simulink model "mcb_pmsm_foc_sensorless_dyno_f28379d"  (R2024b)
settings: Solver=FixedStepDiscrete  StartTime=0.0  StopTime=6  RelTol=1e-3  EnableMultiTasking=on
InitFcn:
  | mcb_pmsm_foc_sensorless_dyno_f28379d_datascript;
model workspace (MAT data in the model file):
  encoderResolution = 2000
  hallOffset = '0.5'
  indexOffset = 850
  polePairs = '4'
values from neighbouring files (symbols this model uses):
  acceleration = 20000/PU_System_motor1.N_base    [mcb_pmsm_foc_sensorless_dyno_f28379d_datascript.m]    (also in soc_mcb_pmsm_foc_dyno_f28379d_data.m = 20000/PU_System.N_base)
  dataType = 'single'    [mcb_pmsm_foc_sensorless_dyno_f28379d_datascript.m]    (also in soc_mcb_pmsm_foc_dyno_f28379d_data.m)
  inverter_motor1 = mcb_SetInverterParameters('BoostXL-DRV8305')    [mcb_pmsm_foc_sensorless_dyno_f28379d_datascript.m]
  inverter_motor2 = mcb_SetInverterParameters('BoostXL-DRV8305')    [mcb_pmsm_foc_sensorless_dyno_f28379d_datascript.m]
  PI_params_motor1 = mcb.internal.SetControllerParameters(pmsm_motor1,inverter_motor1,PU_System_motor1,T_pwm,2*Ts,Ts_speed)    [mcb_pmsm_foc_sensorless_dyno_f28379d_datascript.m]
  PI_params_motor2 = mcb.internal.SetControllerParameters(pmsm_motor2,inverter_motor2,PU_System_motor2,T_pwm,2*Ts,Ts_speed)    [mcb_pmsm_foc_sensorless_dyno_f28379d_datascript.m]
  pmsm_motor1 = mcb_SetPMSMMotorParameters('Teknic2310P')    [mcb_pmsm_foc_sensorless_dyno_f28379d_datascript.m]
  pmsm_motor2 = mcb_SetPMSMMotorParameters('Teknic2310P')    [mcb_pmsm_foc_sensorless_dyno_f28379d_datascript.m]
  PU_System_motor1 = mcb_SetPUSystem(pmsm_motor1,inverter_motor1)    [mcb_pmsm_foc_sensorless_dyno_f28379d_datascript.m]
  PU_System_motor2 = mcb_SetPUSystem(pmsm_motor2,inverter_motor2)    [mcb_pmsm_foc_sensorless_dyno_f28379d_datascript.m]
  PWM_frequency = 20e3    (= 20000)    [mcb_pmsm_foc_sensorless_dyno_f28379d_datascript.m]    (also in soc_mcb_pmsm_foc_dyno_f28379d_data.m)
  Speed_openLoop_PU = 0.1    [mcb_pmsm_foc_sensorless_dyno_f28379d_datascript.m]    (also in soc_mcb_pmsm_foc_dyno_f28379d_data.m)
  T_Ref_openLoop = 1    [mcb_pmsm_foc_sensorless_dyno_f28379d_datascript.m]    (also in soc_mcb_pmsm_foc_dyno_f28379d_data.m)
  target = mcb_SetProcessorDetails('F28379D',PWM_frequency)    [mcb_pmsm_foc_sensorless_dyno_f28379d_datascript.m]    (also in soc_mcb_pmsm_foc_dyno_f28379d_data.m)
  Ts = T_pwm    (= 5e-05)    [mcb_pmsm_foc_sensorless_dyno_f28379d_datascript.m]    (also in soc_mcb_pmsm_foc_dyno_f28379d_data.m)
  Ts_motor = T_pwm/2    (= 2.5e-05)    [mcb_pmsm_foc_sensorless_dyno_f28379d_datascript.m]    (also in soc_mcb_pmsm_foc_dyno_f28379d_data.m)
  Ts_simulink = T_pwm/2    (= 2.5e-05)    [mcb_pmsm_foc_sensorless_dyno_f28379d_datascript.m]    (also in soc_mcb_pmsm_foc_dyno_f28379d_data.m)
  Ts_speed = 20*Ts    (= 0.001)    [mcb_pmsm_foc_sensorless_dyno_f28379d_datascript.m]    (also in soc_mcb_pmsm_foc_dyno_f28379d_data.m)
undefined symbols (not defined in the file or in its folder): Down, GPTRIP1SEL, GPTRIP2SEL, TZ1, TZ2, Up
libraries: mcbcontrolslib x20, c2802xlib x14, simulink x8, c280xlib x7, c2837xDlib x5, slpidlib x4, mcbpositiondecoderlib x4, svdschedulerlib x3, mcbsensorlessestimatorlib x2, mcbpmsmnonlinearlib x2, autolibpmsmexterior x2, mcbplantlib x2
(part 4 of 4)

== system mcb_pmsm_foc_sensorless_dyno_f28379d/FOC Algorithm Motor 2/Input Scaling/Calculate position and speed/Flux Observer ==
  InputSignals : Inport
  Action Port : ActionPort  ActionPortLabel=case [ 1 ]:
  DC component removal : Subsystem
  Data Store Read1 : DataStoreRead  DataStoreName=Enable  IndexOptions=Index vector (dialog)  Indices=1  OutputSizes=1
  Demux2 : Demux
  Flux Observer : mcbpositiondecoderlib/Flux Observer  MotorSelection=PMSM  DataTypeSelect=off  BlockInputUnit=Per-unit  PerUnitVoltage=PU_System_motor2.V_base  PerUnitCurrent=PU_System_motor2.I_base  PositionSelect=on  FluxSelect=off  TorqueSelect=off  PolePairs=4  StatorResistance=pmsm_motor2.Rs  StatorDAxisInductance=pmsm_motor2.Ld  StatorLeakageInductance=0.0068  RotorLeakageInductance=0.0068  MagnetizingInductance=0.0300  CutoffFreq=3.1863  BlockSampleTime=Ts  ParameterBusInput=off  PositionUnit=Per-unit  PositionDatatype=dataType  FluxUnit=Weber  PerUnitFlux=0.1  FluxDatatype=single  TorqueUnit=Nm  PerUnitTorque=100  TorqueDatatype=single  DataType=0
  IIR Filter : mcbcontrolslib/IIR Filter  VariantControl=Low Pass Filter  VariantSelect=Low-pass  FilterConstantInputType=Specify via dialog  Filter_constant=0.01  advancedSettings=off  Ts=50e-6  cutOff_freq=32.1525
  Logical Operator : Logic  Operator=NOT  IconShape=distinctive  AllPortsSameDT=off  OutDataTypeStr=boolean
  Mux2 : Mux  Inputs=2
  Speed Measurement : mcbpositiondecoderlib/Speed Measurement  PositionUnit=Per unit  PositionScalingDatatype=uint32  SpeedCalculationMode=Time interval for speed calculation  SampleTimeAsync=Ts  MaximumApplicationSpeed=60000  SpeedResolution=5e-6  DelayLength=10  MaximumMeasurableSpeed=59999  MeasurableSpeedResolution=2.794e-05  SpeedUnit=Per unit based on dialog  PerUnitSpeed=PU_System_motor2.N_base  SpeedDataType=dataType
  elect2mech : Gain  Gain=1/pmsm_motor2.p  RndMeth=Simplest  OutDataTypeStr=Inherit: Same as input
  Position/Speed : Outport
  wires:
  InputSignals/1 -> DC component removal/1(SigIN)
  Demux2/1 -> Flux Observer/1
  Demux2/2 -> Flux Observer/2
  Mux2/1 -> Position/Speed/1
  Speed Measurement/1 -> IIR Filter/1
  elect2mech/1 -> Mux2/2
  Demux2/3 -> Flux Observer/3  "Ialpha"
  Demux2/4 -> Flux Observer/4  "Ibeta"
  IIR Filter/1 -> elect2mech/1
  Flux Observer/1 -> Mux2/1, Speed Measurement/1
  Logical Operator/1 -> Flux Observer/5
  Data Store Read1/1 -> Logical Operator/1
  DC component removal/1(SigOUT) -> Demux2/1

== system mcb_pmsm_foc_sensorless_dyno_f28379d/FOC Algorithm Motor 2/Input Scaling/Calculate position and speed/Sliding Mode Observer ==
  InputSignals : Inport
  Action Port : ActionPort  ActionPortLabel=case [ 0 ]:
  Data Store Read1 : DataStoreRead  DataStoreName=Enable  IndexOptions=Index vector (dialog)  Indices=1  OutputSizes=1
  Demux1 : Demux
  Logical Operator : Logic  Operator=NOT  IconShape=distinctive  AllPortsSameDT=off  OutDataTypeStr=boolean
  Mux : Mux  Inputs=2
  Sliding Mode Observer : mcbsensorlessestimatorlib/Sliding Mode Observer  InputUnit=Per-unit  BlkSampleTime=Ts  StatorResistance=pmsm_motor2.Rs  StatorInductance=pmsm_motor2.Ld  MaxApplicationSpeed=pmsm_motor2.N_base  PolePairs=pmsm_motor2.p  MaxStatorVoltage=PU_System_motor2.V_base  MaxStatorCurrent=PU_System_motor2.I_base  DisturbanceObserverGain=smo_motor2.BackEmfObsGain  CurrentObserverGain=smo_motor2.CurrentObsGain  CutoffFreq=smo_motor2.CutoffFreq  PositionUnit=Per unit  PositionDataType=dataType  SpeedUnit=Per unit  PerUnitSpeed=PU_System_motor2.N_base  SpeedDataType=dataType
  Position/Speed : Outport
  wires:
  Mux/1 -> Position/Speed/1
  Demux1/1 -> Sliding Mode Observer/1
  Demux1/2 -> Sliding Mode Observer/2
  Demux1/4 -> Sliding Mode Observer/4  "Ibeta"
  Demux1/3 -> Sliding Mode Observer/3  "Ialpha"
  Sliding Mode Observer/1 -> Mux/1
  Sliding Mode Observer/2 -> Mux/2
  InputSignals/1 -> Demux1/1
  Data Store Read1/1 -> Logical Operator/1
  Logical Operator/1 -> Sliding Mode Observer/5

== system mcb_pmsm_foc_sensorless_dyno_f28379d/Hardware Init/HW_Init/HW_Init (Codegen)/Calibrate ADC offset for motor 1 current sensor ==
  note: Enable ADC offset calibration only when motor is not loaded and not rotating due to external factors
  ADC Calib Enable : Constant  Value=inverter_motor1.ADCOffsetCalibEnable  OutDataTypeStr=Inherit: Inherit via back propagation
  "Calculate ADC Offset " : Subsystem  Priority=1001  TreatAsAtomicUnit=on
  Default ADC Offset : Subsystem  Priority=1001  TreatAsAtomicUnit=on
  NOT : Logic  Operator=NOT  IconShape=distinctive  AllPortsSameDT=off  OutDataTypeStr=boolean
  wires:
  NOT/1 -> Default ADC Offset/Enable
  ADC Calib Enable/1 -> "Calculate ADC Offset "/Enable, NOT/1

== system mcb_pmsm_foc_sensorless_dyno_f28379d/Hardware Init/HW_Init/HW_Init (Codegen)/Calibrate ADC offset for motor 2 current sensor ==
  note: Enable ADC offset calibration only when motor is not loaded and not rotating due to external factors
  ADC Calib Enable : Constant  Value=inverter_motor2.ADCOffsetCalibEnable  OutDataTypeStr=Inherit: Inherit via back propagation
  Calculate ADC Offset : Subsystem  Priority=1001  TreatAsAtomicUnit=on
  Default ADC Offset : Subsystem  Priority=1001  TreatAsAtomicUnit=on
  NOT : Logic  Operator=NOT  IconShape=distinctive  AllPortsSameDT=off  OutDataTypeStr=boolean
  wires:
  ADC Calib Enable/1 -> Calculate ADC Offset/Enable, NOT/1
  NOT/1 -> Default ADC Offset/Enable

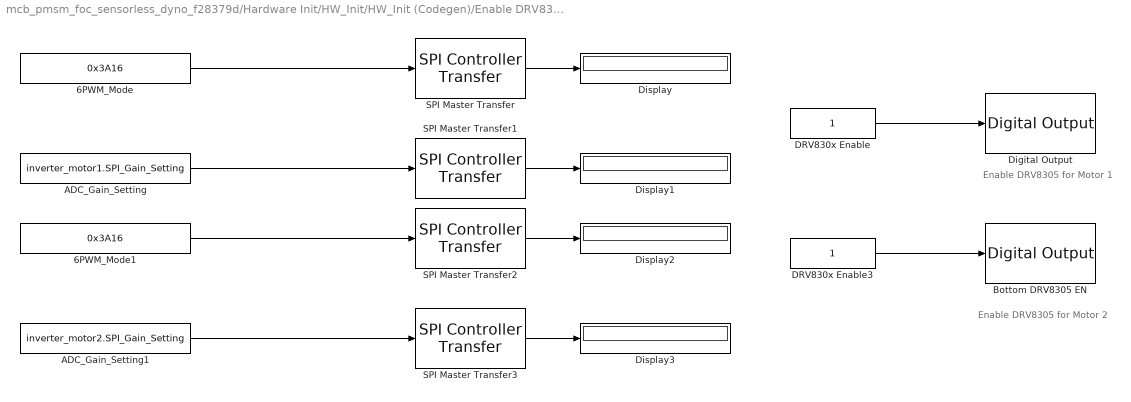
== system mcb_pmsm_foc_sensorless_dyno_f28379d/Hardware Init/HW_Init/HW_Init (Codegen)/Enable DRV8305 for motor 1 and motor 2 ==
  note: Enable DRV8305 for Motor 1
  note: Enable DRV8305 for Motor 2
  6PWM_Mode : Constant  Priority=1000  Value=0x3A16  OutDataTypeStr=uint16  SampleTime=-1
  6PWM_Mode1 : Constant  Priority=1000  Value=0x3A16  OutDataTypeStr=uint16  SampleTime=-1
  ADC_Gain_Setting : Constant  Priority=1000  Value=inverter_motor1.SPI_Gain_Setting  OutDataTypeStr=uint16  SampleTime=-1
  ADC_Gain_Setting1 : Constant  Priority=1000  Value=inverter_motor2.SPI_Gain_Setting  OutDataTypeStr=uint16  SampleTime=-1
  Bottom DRV8305 EN : c2837xDlib/Digital Output  GPIO_Number=GPIO24~GPIO31  GPIO_Bit0=off  GPIO_BIT0_Toggle=off  GPIO_Bit1=off  GPIO_BIT1_Toggle=off  GPIO_Bit2=on  GPIO_BIT2_Toggle=off  GPIO_Bit3=off  GPIO_BIT3_Toggle=off  GPIO_Bit4=off  GPIO_BIT4_Toggle=off  GPIO_Bit5=off  GPIO_BIT5_Toggle=off  GPIO_Bit6=off  GPIO_BIT6_Toggle=off  GPIO_Bit7=off  GPIO_BIT7_Toggle=off
  DRV830x Enable : Constant  OutDataTypeStr=uint16  SampleTime=-1
  DRV830x Enable3 : Constant  OutDataTypeStr=uint16  SampleTime=-1
  Digital Output : c2837xDlib/Digital Output  Priority=10  GPIO_Number=GPIO120~GPIO127  GPIO_Bit0=off  GPIO_BIT0_Toggle=off  GPIO_Bit1=off  GPIO_BIT1_Toggle=off  GPIO_Bit2=off  GPIO_BIT2_Toggle=off  GPIO_Bit3=off  GPIO_BIT3_Toggle=off  GPIO_Bit4=on  GPIO_BIT4_Toggle=off  GPIO_Bit5=off  GPIO_BIT5_Toggle=off  GPIO_Bit6=off  GPIO_BIT6_Toggle=off  GPIO_Bit7=off  GPIO_BIT7_Toggle=off
  Display{,1..3} (4 alike) : Display
      settings: Format=hex (Stored Integer)
  SPI Master Transfer : c280xlib/SPI Controller Transfer  SPISelect=SPI_A  ClockPolarity=Rising_edge  ClockPhase=No_delay  SPIModule=uint32(0)  Mode=Master  BusSpeed=uint32(1000000)  FirstBitToTransfer=Most significant bit (MSB)  ClockMode=0  BlockFunction=Transfer  EnableRegisterAddress=off  RegisterAddress=0  OutputDataType=int8  OutputDataLength=1  DataBits=16  UseCustomSSPin=Provided by the SPI peripheral  ActiveLowSSPin=Active low  Pin=61
  SPI Master Transfer1 : c280xlib/SPI Controller Transfer  SPISelect=SPI_A  ClockPolarity=Rising_edge  ClockPhase=No_delay  SPIModule=uint32(0)  Mode=Master  BusSpeed=uint32(1000000)  FirstBitToTransfer=Most significant bit (MSB)  ClockMode=0  BlockFunction=Transfer  EnableRegisterAddress=off  RegisterAddress=0  OutputDataType=int8  OutputDataLength=1  DataBits=16  UseCustomSSPin=Provided by the SPI peripheral  ActiveLowSSPin=Active low  Pin=61
  SPI Master Transfer2 : c280xlib/SPI Controller Transfer  SPISelect=SPI_B  ClockPolarity=Rising_edge  ClockPhase=No_delay  SPIModule=uint32(0)  Mode=Master  BusSpeed=uint32(1000000)  FirstBitToTransfer=Most significant bit (MSB)  ClockMode=0  BlockFunction=Transfer  EnableRegisterAddress=off  RegisterAddress=0  OutputDataType=int8  OutputDataLength=1  DataBits=16  UseCustomSSPin=Provided by the SPI peripheral  ActiveLowSSPin=Active low  Pin=61
  SPI Master Transfer3 : c280xlib/SPI Controller Transfer  SPISelect=SPI_B  ClockPolarity=Rising_edge  ClockPhase=No_delay  SPIModule=uint32(0)  Mode=Master  BusSpeed=uint32(1000000)  FirstBitToTransfer=Most significant bit (MSB)  ClockMode=0  BlockFunction=Transfer  EnableRegisterAddress=off  RegisterAddress=0  OutputDataType=int8  OutputDataLength=1  DataBits=16  UseCustomSSPin=Provided by the SPI peripheral  ActiveLowSSPin=Active low  Pin=61
  wires:
  DRV830x Enable/1 -> Digital Output/1
  DRV830x Enable3/1 -> Bottom DRV8305 EN/1
  6PWM_Mode1/1 -> SPI Master Transfer2/1
  6PWM_Mode/1 -> SPI Master Transfer/1
  ADC_Gain_Setting/1 -> SPI Master Transfer1/1
  SPI Master Transfer3/1 -> Display3/1
  SPI Master Transfer2/1 -> Display2/1
  SPI Master Transfer1/1 -> Display1/1
  SPI Master Transfer/1 -> Display/1
  ADC_Gain_Setting1/1 -> SPI Master Transfer3/1

== system mcb_pmsm_foc_sensorless_dyno_f28379d/Serial Receive/Parse SCI Rx/Data_Conditioning_Rx/Data_Type_Fixed_Point ==
  Rx : Inport
  Data Type Conversion1 : DataTypeConversion  OutDataTypeStr=dataType  RndMeth=Simplest  SaturateOnIntegerOverflow=off
  Data Type Conversion2 : DataTypeConversion  OutDataTypeStr=fixdt(1,32,28)  ConvertRealWorld=Stored Integer (SI)  RndMeth=Simplest  SaturateOnIntegerOverflow=off
  Data Type Conversion3 : DataTypeConversion  OutDataTypeStr=uint16  RndMeth=Simplest  SaturateOnIntegerOverflow=off
  Data Type Conversion4 : DataTypeConversion  OutDataTypeStr=dataType  RndMeth=Simplest  SaturateOnIntegerOverflow=off
  Data Type Conversion5 : DataTypeConversion  OutDataTypeStr=fixdt(1,32,28)  ConvertRealWorld=Stored Integer (SI)  RndMeth=Simplest  SaturateOnIntegerOverflow=off
  Demux : Demux  Outputs=3
  Desired Speed : Outport
  Out2 : Outport  Port=2
  Desired torque : Outport  Port=3
  wires:
  Rx/1 -> Demux/1
  Data Type Conversion1/1 -> Desired Speed/1
  Data Type Conversion2/1 -> Data Type Conversion1/1
  Demux/1 -> Data Type Conversion2/1
  Demux/2 -> Data Type Conversion3/1
  Data Type Conversion3/1 -> Out2/1
  Demux/3 -> Data Type Conversion5/1
  Data Type Conversion5/1 -> Data Type Conversion4/1
  Data Type Conversion4/1 -> Desired torque/1

== system mcb_pmsm_foc_sensorless_dyno_f28379d/Serial Receive/Parse SCI Rx/Data_Conditioning_Rx/Data_Type_Float ==
  Rx : Inport
  Data Type Conversion2 : DataTypeConversion  OutDataTypeStr=uint16  RndMeth=Simplest  SaturateOnIntegerOverflow=off
  Demux : Demux  Outputs=3
  Desired Speed : Outport
  Out2 : Outport  Port=2
  Desired torque : Outport  Port=3
  wires:
  Rx/1 -> Demux/1
  Demux/1 -> Desired Speed/1
  Data Type Conversion2/1 -> Out2/1
  Demux/2 -> Data Type Conversion2/1
  Demux/3 -> Desired torque/1

== system mcb_pmsm_foc_sensorless_dyno_f28379d/Serial Receive/Serial Receive/Serial Rx/Data_Type_Fixed_Point ==
  SCI Receive : c280xlib/SCI Receive  sciModule=A  dataHead=''  headerCheckMaxCount=16  dataTail=''  dataType=uint32  dataLenOptions=Length via dialog  dataDim=3  maxDataLength=1  initValue=0  errOption=Output the last received value  errValue=0  sampleTime=-1  blockingMode=on  timeOut=0.00875  outputStatus=off
  Rx : Outport
  wires:
  SCI Receive/1 -> Rx/1

== system mcb_pmsm_foc_sensorless_dyno_f28379d/Serial Receive/Serial Receive/Serial Rx/Data_Type_Float ==
  SCI Receive : c280xlib/SCI Receive  sciModule=A  dataHead=''  headerCheckMaxCount=16  dataTail=''  dataType=single  dataLenOptions=Length via dialog  dataDim=3  maxDataLength=1  initValue=0  errOption=Output the last received value  errValue=0  sampleTime=-1  blockingMode=on  timeOut=0.00875  outputStatus=off
  Rx : Outport
  wires:
  SCI Receive/1 -> Rx/1

== system mcb_pmsm_foc_sensorless_dyno_f28379d/Serial Receive/Signal Packing/Data_Conditioning_Tx/Data_Type_Fixed_Point ==
  In1 : Inport
  In2 : Inport  Port=2
  In3 : Inport  Port=3
  Data Type Conversion : DataTypeConversion  OutDataTypeStr=fixdt(1,32,28)  RndMeth=Simplest  SaturateOnIntegerOverflow=off
  Data Type Conversion1 : DataTypeConversion  OutDataTypeStr=uint32  RndMeth=Simplest  SaturateOnIntegerOverflow=off
  Data Type Conversion2 : DataTypeConversion  OutDataTypeStr=fixdt(1,32,28)  RndMeth=Simplest  SaturateOnIntegerOverflow=off
  Data Type Conversion3 : DataTypeConversion  OutDataTypeStr=uint32  ConvertRealWorld=Stored Integer (SI)  RndMeth=Simplest  SaturateOnIntegerOverflow=off
  Data Type Conversion4 : DataTypeConversion  OutDataTypeStr=uint32  ConvertRealWorld=Stored Integer (SI)  RndMeth=Simplest  SaturateOnIntegerOverflow=off
  Mux : Mux  Inputs=3
  Data : Outport
  wires:
  In1/1 -> Data Type Conversion/1
  Data Type Conversion3/1 -> Mux/1
  Data Type Conversion/1 -> Data Type Conversion3/1
  In2/1 -> Data Type Conversion1/1
  Data Type Conversion1/1 -> Mux/2
  Mux/1 -> Data/1
  Data Type Conversion2/1 -> Data Type Conversion4/1
  Data Type Conversion4/1 -> Mux/3
  In3/1 -> Data Type Conversion2/1

== system mcb_pmsm_foc_sensorless_dyno_f28379d/Serial Receive/Signal Packing/Data_Conditioning_Tx/Data_Type_Float ==
  In1 : Inport
  In2 : Inport  Port=2
  In3 : Inport  Port=3
  Data Type Conversion2 : DataTypeConversion  OutDataTypeStr=single  RndMeth=Simplest  SaturateOnIntegerOverflow=off
  Mux : Mux  Inputs=3
  Data : Outport
  wires:
  In1/1 -> Mux/1
  Mux/1 -> Data/1
  In2/1 -> Data Type Conversion2/1
  Data Type Conversion2/1 -> Mux/2
  In3/1 -> Mux/3

== system mcb_pmsm_foc_sensorless_dyno_f28379d/FOC Algorithm Motor 1/Input Scaling/Calculate Phase Currents/Data_Type/Data_Type_Fixed_Point ==
  In1 : Inport
  Data Type Conversion : DataTypeConversion  OutDataTypeStr=fixdt(1,32,17)  ConvertRealWorld=Stored Integer (SI)  RndMeth=Simplest  SaturateOnIntegerOverflow=off
  Data Type Conversion1 : DataTypeConversion  OutDataTypeStr=dataType  RndMeth=Simplest  SaturateOnIntegerOverflow=off
  Q17 per unit conversion : ArithShift  BitShiftNumber=-6
  Iab_meas_PU : Outport
  wires:
  In1/1 -> Q17 per unit conversion/1
  Data Type Conversion1/1 -> Iab_meas_PU/1
  Data Type Conversion/1 -> Data Type Conversion1/1
  Q17 per unit conversion/1 -> Data Type Conversion/1

== system mcb_pmsm_foc_sensorless_dyno_f28379d/FOC Algorithm Motor 1/Input Scaling/Calculate Phase Currents/Data_Type/Data_Type_Float ==
  In1 : Inport
  Get ADC Voltage : Gain  Gain=target.ADC_Vref /target.ADC_MaxCount  OutDataTypeStr=dataType  RndMeth=Simplest
  Get Currents : Gain  Gain=1/inverter_motor1.ISenseVoltPerAmp  RndMeth=Simplest  OutDataTypeStr=Inherit: Same as input
  PU_Conversion : Gain  Gain=1/PU_System_motor1.I_base  RndMeth=Simplest  OutDataTypeStr=Inherit: Same as input
  Iab_meas_PU : Outport
  wires:
  Get ADC Voltage/1 -> Get Currents/1
  Get Currents/1 -> PU_Conversion/1
  PU_Conversion/1 -> Iab_meas_PU/1
  In1/1 -> Get ADC Voltage/1

== system mcb_pmsm_foc_sensorless_dyno_f28379d/FOC Algorithm Motor 1/Input Scaling/Calculate position and speed/Flux Observer/DC component removal ==
  SigIN : Inport
  IIR Filter : mcbcontrolslib/IIR Filter  VariantControl=Low Pass Filter  VariantSelect=Low-pass  FilterConstantInputType=Specify via dialog  Filter_constant=0.005*(Ts/50e-6)  advancedSettings=off  Ts=50e-6  cutOff_freq=15.9955
  Sum6 : Sum  Inputs=|+-  RndMeth=Simplest  OutDataTypeStr=Inherit: Same as first input
  SigOUT : Outport
  wires:
  IIR Filter/1 -> Sum6/2
  SigIN/1 -> IIR Filter/1, Sum6/1
  Sum6/1 -> SigOUT/1

== system mcb_pmsm_foc_sensorless_dyno_f28379d/FOC Algorithm Motor 2/Enable Motor2 after a delay/Delay to start motor2 (codegen)/Enable EnMtr2TrqCtrl after 2 sec delay/Enable EnMtr2TrqCtrl ==
  Enable : EnablePort  StatesWhenEnabling=reset
  Constant : Constant  OutDataTypeStr=boolean
  Data Store Write : DataStoreWrite  DataStoreName=EnMtr2TrqCtrl  IndexOptions=Index vector (dialog)  Indices=1  OutputSizes=1
  wires:
  Constant/1 -> Data Store Write/1

== system mcb_pmsm_foc_sensorless_dyno_f28379d/FOC Algorithm Motor 2/Input Scaling/Calculate Phase Currents/Data_Type/Data_Type_Fixed_Point ==
  In1 : Inport
  Data Type Conversion : DataTypeConversion  OutDataTypeStr=fixdt(1,32,17)  ConvertRealWorld=Stored Integer (SI)  RndMeth=Simplest  SaturateOnIntegerOverflow=off
  Data Type Conversion1 : DataTypeConversion  OutDataTypeStr=dataType  RndMeth=Simplest  SaturateOnIntegerOverflow=off
  Q17 per unit conversion : ArithShift  BitShiftNumber=-6
  Iab_meas_PU : Outport
  wires:
  Q17 per unit conversion/1 -> Data Type Conversion/1
  Data Type Conversion/1 -> Data Type Conversion1/1
  Data Type Conversion1/1 -> Iab_meas_PU/1
  In1/1 -> Q17 per unit conversion/1

== system mcb_pmsm_foc_sensorless_dyno_f28379d/FOC Algorithm Motor 2/Input Scaling/Calculate Phase Currents/Data_Type/Data_Type_Float ==
  In1 : Inport
  Get ADC Voltage : Gain  Gain=target.ADC_Vref /target.ADC_MaxCount  OutDataTypeStr=dataType  RndMeth=Simplest
  Get Currents : Gain  Gain=1/inverter_motor2.ISenseVoltPerAmp  RndMeth=Simplest  OutDataTypeStr=Inherit: Same as input
  PU_Conversion : Gain  Gain=1/PU_System_motor2.I_base  RndMeth=Simplest  OutDataTypeStr=Inherit: Same as input
  Iab_meas_PU : Outport
  wires:
  Get ADC Voltage/1 -> Get Currents/1
  Get Currents/1 -> PU_Conversion/1
  PU_Conversion/1 -> Iab_meas_PU/1
  In1/1 -> Get ADC Voltage/1

== system mcb_pmsm_foc_sensorless_dyno_f28379d/FOC Algorithm Motor 2/Input Scaling/Calculate position and speed/Flux Observer/DC component removal ==
  SigIN : Inport
  IIR Filter : mcbcontrolslib/IIR Filter  VariantControl=Low Pass Filter  VariantSelect=Low-pass  FilterConstantInputType=Specify via dialog  Filter_constant=0.005*(Ts/50e-6)  advancedSettings=off  Ts=50e-6  cutOff_freq=15.9955
  Sum6 : Sum  Inputs=|+-  RndMeth=Simplest  OutDataTypeStr=Inherit: Same as first input
  SigOUT : Outport
  wires:
  IIR Filter/1 -> Sum6/2
  SigIN/1 -> IIR Filter/1, Sum6/1
  Sum6/1 -> SigOUT/1

== system mcb_pmsm_foc_sensorless_dyno_f28379d/Hardware Init/HW_Init/HW_Init (Codegen)/Calibrate ADC offset for motor 1 current sensor/Calculate ADC Offset  ==
  Enable : EnablePort
  Constant : Constant  Value=8
  Constant1 : Constant  Value=inverter_motor1.CtSensOffsetMax  OutDataTypeStr=Inherit: Inherit via back propagation
  Constant2 : Constant  Value=inverter_motor1.CtSensOffsetMin  OutDataTypeStr=Inherit: Inherit via back propagation
  Divide : Product  Inputs=*/  OutDataTypeStr=uint16
  Divide1 : Product  Inputs=*/  OutDataTypeStr=uint16
  For Iterator Subsystem : Subsystem  TreatAsAtomicUnit=on
  If : If  NumInputs=3  IfExpression=u1 > u3 & u1 < u2
  If Action Subsystem : Subsystem  TreatAsAtomicUnit=on
  If Action Subsystem1 : Subsystem  TreatAsAtomicUnit=on
  If Action Subsystem2 : Subsystem  TreatAsAtomicUnit=on
  If Action Subsystem3 : Subsystem  TreatAsAtomicUnit=on
  If1 : If  NumInputs=3  IfExpression=u1 > u3 & u1 < u2
  wires:
  For Iterator Subsystem/2(Out2) -> Divide1/1
  Divide/1 -> If Action Subsystem/1(In1), If/1
  For Iterator Subsystem/1(Out1) -> Divide/1
  Constant/1 -> Divide/2, Divide1/2
  Divide1/1 -> If1/1, If Action Subsystem2/1(In1)
  If/1 -> If Action Subsystem/Action
  If/2 -> If Action Subsystem1/Action
  If1/1 -> If Action Subsystem2/Action
  If1/2 -> If Action Subsystem3/Action
  Constant1/1 -> If/2, If1/2
  Constant2/1 -> If/3, If1/3

== system mcb_pmsm_foc_sensorless_dyno_f28379d/Hardware Init/HW_Init/HW_Init (Codegen)/Calibrate ADC offset for motor 1 current sensor/Default ADC Offset ==
  Enable : EnablePort
  Constant : Constant  Value=inverter_motor1.CtSensAOffset  OutDataTypeStr=Inherit: Inherit via back propagation
  Constant1 : Constant  Value=inverter_motor1.CtSensBOffset  OutDataTypeStr=Inherit: Inherit via back propagation
  Data Store Write1 : DataStoreWrite  DataStoreName=IaOffset_motor1  IndexOptions=Index vector (dialog)  Indices=1  OutputSizes=1
  Data Store Write2 : DataStoreWrite  DataStoreName=IbOffset_motor1  IndexOptions=Index vector (dialog)  Indices=1  OutputSizes=1
  wires:
  Constant/1 -> Data Store Write1/1
  Constant1/1 -> Data Store Write2/1

== system mcb_pmsm_foc_sensorless_dyno_f28379d/Hardware Init/HW_Init/HW_Init (Codegen)/Calibrate ADC offset for motor 2 current sensor/Calculate ADC Offset ==
  Enable : EnablePort
  Constant1 : Constant  Value=8
  Constant2 : Constant  Value=inverter_motor2.CtSensOffsetMax  OutDataTypeStr=Inherit: Inherit via back propagation
  Constant3 : Constant  Value=inverter_motor2.CtSensOffsetMin  OutDataTypeStr=Inherit: Inherit via back propagation
  Divide2 : Product  Inputs=*/  OutDataTypeStr=uint16
  Divide3 : Product  Inputs=*/  OutDataTypeStr=uint16
  For Iterator Subsystem : Subsystem  TreatAsAtomicUnit=on
  If Action Subsystem4 : Subsystem  TreatAsAtomicUnit=on
  If Action Subsystem5 : Subsystem  TreatAsAtomicUnit=on
  If Action Subsystem6 : Subsystem  TreatAsAtomicUnit=on
  If Action Subsystem7 : Subsystem  TreatAsAtomicUnit=on
  If2 : If  NumInputs=3  IfExpression=u1 > u3 & u1 < u2
  If3 : If  NumInputs=3  IfExpression=u1 > u3 & u1 < u2
  wires:
  For Iterator Subsystem/2(Out4) -> Divide3/1
  Divide2/1 -> If2/1, If Action Subsystem4/1(In1)
  For Iterator Subsystem/1(Out3) -> Divide2/1
  Constant1/1 -> Divide2/2, Divide3/2
  Divide3/1 -> If3/1, If Action Subsystem6/1(In1)
  If2/1 -> If Action Subsystem4/Action
  If2/2 -> If Action Subsystem5/Action
  If3/1 -> If Action Subsystem6/Action
  If3/2 -> If Action Subsystem7/Action
  Constant2/1 -> If2/2, If3/2
  Constant3/1 -> If2/3, If3/3

== system mcb_pmsm_foc_sensorless_dyno_f28379d/Hardware Init/HW_Init/HW_Init (Codegen)/Calibrate ADC offset for motor 2 current sensor/Default ADC Offset ==
  Enable : EnablePort
  Constant2 : Constant  Value=inverter_motor2.CtSensAOffset  OutDataTypeStr=Inherit: Inherit via back propagation
  Constant3 : Constant  Value=inverter_motor2.CtSensBOffset  OutDataTypeStr=Inherit: Inherit via back propagation
  Data Store Write3 : DataStoreWrite  DataStoreName=IaOffset_motor2  IndexOptions=Index vector (dialog)  Indices=1  OutputSizes=1
  Data Store Write4 : DataStoreWrite  DataStoreName=IbOffset_motor2  IndexOptions=Index vector (dialog)  Indices=1  OutputSizes=1
  wires:
  Constant2/1 -> Data Store Write3/1
  Constant3/1 -> Data Store Write4/1

== system mcb_pmsm_foc_sensorless_dyno_f28379d/Hardware Init/HW_Init/HW_Init (Codegen)/Calibrate ADC offset for motor 1 current sensor/Calculate ADC Offset /For Iterator Subsystem ==
  ADC_A_IN0 : c2802xlib/ADC  Priority=20  blkParamProc=C2000_Type4  ADCModule=C  samplingMode=Single sample mode  ADCResolution=12-bit (Single-ended input)  useSOC1=SOC2  useSOC2=SOC0_SOC1  SOCAcquisitionWindow=15  SOCTriggerSource=Software  SOCInterruptTrigger=No ADCINT  Ts=-1  dType=uint16  postInterrupt=off  interruptSel=ADCINT1  ADCINTContinuous=on  endma=off  chdma=1  conv1=ADCINA0  conv2=ADCINA0 and ADCINB0  conv1_Type4=ADCIN2  conv2_Type4=ADCIN0 and ADCIN1
  ADC_B_IN0 : c2802xlib/ADC  Priority=20  blkParamProc=C2000_Type4  ADCModule=B  samplingMode=Single sample mode  ADCResolution=12-bit (Single-ended input)  useSOC1=SOC2  useSOC2=SOC0_SOC1  SOCAcquisitionWindow=15  SOCTriggerSource=Software  SOCInterruptTrigger=No ADCINT  Ts=-1  dType=uint16  postInterrupt=off  interruptSel=ADCINT1  ADCINTContinuous=on  endma=off  chdma=1  conv1=ADCINA0  conv2=ADCINA0 and ADCINB0  conv1_Type4=ADCIN2  conv2_Type4=ADCIN0 and ADCIN1
  For Iterator : ForIterator  IterationLimit=16  IterationVariableDataType=uint16
  If : If  IfExpression=u1 > 8  ShowElse=off
  If Action Subsystem : Subsystem  TreatAsAtomicUnit=on
  Out1 : Outport
  Out2 : Outport  Port=2
  wires:
  For Iterator/1 -> If/1
  ADC_A_IN0/1 -> If Action Subsystem/1(In1)
  ADC_B_IN0/1 -> If Action Subsystem/2(In2)
  If Action Subsystem/1(Out1) -> Out1/1
  If Action Subsystem/2(Out2) -> Out2/1
  If/1 -> If Action Subsystem/Action

== system mcb_pmsm_foc_sensorless_dyno_f28379d/Hardware Init/HW_Init/HW_Init (Codegen)/Calibrate ADC offset for motor 1 current sensor/Calculate ADC Offset /If Action Subsystem ==
  In1 : Inport
  Action Port : ActionPort  ActionPortLabel=if(u1 > u3 & u1 < u2)
  Data Store Write1 : DataStoreWrite  DataStoreName=IaOffset_motor1  IndexOptions=Index vector (dialog)  Indices=1  OutputSizes=1
  wires:
  In1/1 -> Data Store Write1/1

== system mcb_pmsm_foc_sensorless_dyno_f28379d/Hardware Init/HW_Init/HW_Init (Codegen)/Calibrate ADC offset for motor 1 current sensor/Calculate ADC Offset /If Action Subsystem1 ==
  Action Port : ActionPort  ActionPortLabel=else
  Constant : Constant  Value=inverter_motor1.CtSensAOffset  OutDataTypeStr=Inherit: Inherit via back propagation
  Data Store Write1 : DataStoreWrite  DataStoreName=IaOffset_motor1  IndexOptions=Index vector (dialog)  Indices=1  OutputSizes=1
  wires:
  Constant/1 -> Data Store Write1/1

== system mcb_pmsm_foc_sensorless_dyno_f28379d/Hardware Init/HW_Init/HW_Init (Codegen)/Calibrate ADC offset for motor 1 current sensor/Calculate ADC Offset /If Action Subsystem2 ==
  In1 : Inport
  Action Port : ActionPort  ActionPortLabel=if(u1 > u3 & u1 < u2)
  Data Store Write2 : DataStoreWrite  DataStoreName=IbOffset_motor1  IndexOptions=Index vector (dialog)  Indices=1  OutputSizes=1
  wires:
  In1/1 -> Data Store Write2/1

== system mcb_pmsm_foc_sensorless_dyno_f28379d/Hardware Init/HW_Init/HW_Init (Codegen)/Calibrate ADC offset for motor 1 current sensor/Calculate ADC Offset /If Action Subsystem3 ==
  Action Port : ActionPort  ActionPortLabel=else
  Constant1 : Constant  Value=inverter_motor1.CtSensBOffset  OutDataTypeStr=Inherit: Inherit via back propagation
  Data Store Write2 : DataStoreWrite  DataStoreName=IbOffset_motor1  IndexOptions=Index vector (dialog)  Indices=1  OutputSizes=1
  wires:
  Constant1/1 -> Data Store Write2/1

== system mcb_pmsm_foc_sensorless_dyno_f28379d/Hardware Init/HW_Init/HW_Init (Codegen)/Calibrate ADC offset for motor 2 current sensor/Calculate ADC Offset/For Iterator Subsystem ==
  ADC_A_IN1 : c2802xlib/ADC  Priority=20  blkParamProc=C2000_Type4  ADCModule=C  samplingMode=Single sample mode  ADCResolution=12-bit (Single-ended input)  useSOC1=SOC3  useSOC2=SOC0_SOC1  SOCAcquisitionWindow=15  SOCTriggerSource=Software  SOCInterruptTrigger=No ADCINT  Ts=-1  dType=uint16  postInterrupt=off  interruptSel=ADCINT1  ADCINTContinuous=on  endma=off  chdma=1  conv1=ADCINA0  conv2=ADCINA0 and ADCINB0  conv1_Type4=ADCIN4  conv2_Type4=ADCIN0 and ADCIN1
  ADC_B_IN1 : c2802xlib/ADC  Priority=20  blkParamProc=C2000_Type4  ADCModule=B  samplingMode=Single sample mode  ADCResolution=12-bit (Single-ended input)  useSOC1=SOC3  useSOC2=SOC0_SOC1  SOCAcquisitionWindow=15  SOCTriggerSource=Software  SOCInterruptTrigger=No ADCINT  Ts=-1  dType=uint16  postInterrupt=off  interruptSel=ADCINT1  ADCINTContinuous=on  endma=off  chdma=1  conv1=ADCINA0  conv2=ADCINA0 and ADCINB0  conv1_Type4=ADCIN4  conv2_Type4=ADCIN0 and ADCIN1
  For Iterator : ForIterator  IterationLimit=16  IterationVariableDataType=uint16
  If Action Subsystem1 : Subsystem  TreatAsAtomicUnit=on
  If1 : If  IfExpression=u1 > 8  ShowElse=off
  Out3 : Outport
  Out4 : Outport  Port=2
  wires:
  If1/1 -> If Action Subsystem1/Action
  If Action Subsystem1/2(Out2) -> Out4/1
  If Action Subsystem1/1(Out1) -> Out3/1
  ADC_B_IN1/1 -> If Action Subsystem1/2(In2)
  ADC_A_IN1/1 -> If Action Subsystem1/1(In1)
  For Iterator/1 -> If1/1

== system mcb_pmsm_foc_sensorless_dyno_f28379d/Hardware Init/HW_Init/HW_Init (Codegen)/Calibrate ADC offset for motor 2 current sensor/Calculate ADC Offset/If Action Subsystem4 ==
  In1 : Inport
  Action Port : ActionPort  ActionPortLabel=if(u1 > u3 & u1 < u2)
  Data Store Write1 : DataStoreWrite  DataStoreName=IaOffset_motor2  IndexOptions=Index vector (dialog)  Indices=1  OutputSizes=1
  wires:
  In1/1 -> Data Store Write1/1

== system mcb_pmsm_foc_sensorless_dyno_f28379d/Hardware Init/HW_Init/HW_Init (Codegen)/Calibrate ADC offset for motor 2 current sensor/Calculate ADC Offset/If Action Subsystem5 ==
  Action Port : ActionPort  ActionPortLabel=else
  Constant : Constant  Value=inverter_motor2.CtSensAOffset  OutDataTypeStr=Inherit: Inherit via back propagation
  Data Store Write1 : DataStoreWrite  DataStoreName=IaOffset_motor2  IndexOptions=Index vector (dialog)  Indices=1  OutputSizes=1
  wires:
  Constant/1 -> Data Store Write1/1

== system mcb_pmsm_foc_sensorless_dyno_f28379d/Hardware Init/HW_Init/HW_Init (Codegen)/Calibrate ADC offset for motor 2 current sensor/Calculate ADC Offset/If Action Subsystem6 ==
  In1 : Inport
  Action Port : ActionPort  ActionPortLabel=if(u1 > u3 & u1 < u2)
  Data Store Write2 : DataStoreWrite  DataStoreName=IbOffset_motor2  IndexOptions=Index vector (dialog)  Indices=1  OutputSizes=1
  wires:
  In1/1 -> Data Store Write2/1

== system mcb_pmsm_foc_sensorless_dyno_f28379d/Hardware Init/HW_Init/HW_Init (Codegen)/Calibrate ADC offset for motor 2 current sensor/Calculate ADC Offset/If Action Subsystem7 ==
  Action Port : ActionPort  ActionPortLabel=else
  Constant1 : Constant  Value=inverter_motor2.CtSensBOffset  OutDataTypeStr=Inherit: Inherit via back propagation
  Data Store Write2 : DataStoreWrite  DataStoreName=IbOffset_motor2  IndexOptions=Index vector (dialog)  Indices=1  OutputSizes=1
  wires:
  Constant1/1 -> Data Store Write2/1

== system mcb_pmsm_foc_sensorless_dyno_f28379d/Hardware Init/HW_Init/HW_Init (Codegen)/Calibrate ADC offset for motor 1 current sensor/Calculate ADC Offset /For Iterator Subsystem/If Action Subsystem ==
  In1 : Inport
  In2 : Inport  Port=2
  Action Port : ActionPort  ActionPortLabel=if(u1 > 8)
  Memory : Memory  InheritSampleTime=on
  Memory1 : Memory  InheritSampleTime=on
  Sum : Sum
  Sum1 : Sum
  Out1 : Outport
  Out2 : Outport  Port=2
  wires:
  In1/1 -> Sum/1
  Sum/1 -> Out1/1, Memory/1
  In2/1 -> Sum1/1
  Memory/1 -> Sum/2
  Sum1/1 -> Out2/1, Memory1/1
  Memory1/1 -> Sum1/2

== system mcb_pmsm_foc_sensorless_dyno_f28379d/Hardware Init/HW_Init/HW_Init (Codegen)/Calibrate ADC offset for motor 2 current sensor/Calculate ADC Offset/For Iterator Subsystem/If Action Subsystem1 ==
  In1 : Inport
  In2 : Inport  Port=2
  Action Port : ActionPort  ActionPortLabel=if(u1 > 8)
  Memory : Memory  InheritSampleTime=on
  Memory1 : Memory  InheritSampleTime=on
  Sum : Sum
  Sum1 : Sum
  Out1 : Outport
  Out2 : Outport  Port=2
  wires:
  In1/1 -> Sum/1
  Sum/1 -> Out1/1, Memory/1
  In2/1 -> Sum1/1
  Memory/1 -> Sum/2
  Sum1/1 -> Out2/1, Memory1/1
  Memory1/1 -> Sum1/2

== matlab function mcb_pmsm_foc_sensorless_dyno_f28379d/FOC Algorithm Motor 1/Closed Loop/Current_Controllers/PI_Controller_Id/PI_Controller_Id ==
  data: e input; V_d_ref output; P input; I_Ts_speed input; reset input; Id0 input; saturation_limit input
function V_d_ref = PI_Controller(e, P, I_Ts_speed, reset, Id0, saturation_limit)
    % PI_Controller: implementa un controllore PI con saturazione e reset.
    % INPUTS:
    % e               -> Errore (input del PI)
    % P               -> Guadagno proporzionale
    % I_Ts_speed      -> Guadagno integrale moltiplicato per Ts (I*Ts_speed)
    % reset           -> Segnale booleano per resettare l'integratore
    % Id0              -> Valore iniziale del riferimento (per l'integratore)
    % saturation_limit -> Limite di saturazione (valore assoluto)
    %
    % OUTPUT:
    % V_d_ref         -> Uscita del controllore PI con saturazione
    
    % Definizione di variabili statiche per la memoria interna del PI
    persistent integrator_state;
    if isempty(integrator_state)
        integrator_state = single(0);  % Inizializza la memoria dell'integratore
    end
    
    % Reset integratore se richiesto
    if reset
        integrator_state = Id0;
    end
    
    % Parte proporzionale
    P_term = P * e;
    
    % Parte integrale (accumulatore)
    integrator_state = integrator_state + I_Ts_speed * e;
    
    % Uscita PI senza saturazione
    V_d_ref_unsat = P_term + integrator_state;
    
    % Saturazione dell'uscita (limite superiore e inferiore)
    V_d_ref = max(min(V_d_ref_unsat, saturation_limit), -saturation_limit);
    
    % Implementazione dell'anti-windup: corregge l'integratore in caso di saturazione
    if V_d_ref ~= V_d_ref_unsat
        integrator_state = integrator_state - I_Ts_speed * e;  % Evita windup
    end
end

== matlab function mcb_pmsm_foc_sensorless_dyno_f28379d/Speed Control/PI_Controller_Speed/PI_Controller_Speed ==
  data: e input; Trq_ref output; P input; I_Ts_speed input; reset input; I0 input; saturation_limit input
function Trq_ref = PI_Controller(e, P, I_Ts_speed, reset, I0, saturation_limit)
    % PI_Controller: implementa un controllore PI con saturazione e reset.
    % INPUTS:
    % e               -> Errore (input del PI)
    % P               -> Guadagno proporzionale
    % I_Ts_speed      -> Guadagno integrale moltiplicato per Ts (I*Ts_speed)
    % reset           -> Segnale booleano per resettare l'integratore
    % I0              -> Valore iniziale del riferimento (per l'integratore)
    % saturation_limit -> Limite di saturazione (valore assoluto)
    %
    % OUTPUT:
    % Trq_ref         -> Uscita del controllore PI con saturazione
    
    % Definizione di variabili statiche per la memoria interna del PI
    persistent integrator_state;
    if isempty(integrator_state)
        integrator_state = single(0);  % Inizializza la memoria dell'integratore
    end
    
    % Reset integratore se richiesto
    if reset
        integrator_state = I0;
    end
    
    % Parte proporzionale
    P_term = P * e;
    
    % Parte integrale (accumulatore)
    integrator_state = integrator_state + I_Ts_speed * e;
    
    % Uscita PI senza saturazione
    Trq_ref_unsat = P_term + integrator_state;
    
    % Saturazione dell'uscita (limite superiore e inferiore)
    Trq_ref = max(min(Trq_ref_unsat, saturation_limit), -saturation_limit);
    
    % Implementazione dell'anti-windup: corregge l'integratore in caso di saturazione
    if Trq_ref ~= Trq_ref_unsat
        integrator_state = integrator_state - I_Ts_speed * e;  % Evita windup
    end
end

== matlab function mcb_pmsm_foc_sensorless_dyno_f28379d/FOC Algorithm Motor 2/Closed loop/Current_Controllers/PI_Controller_Id/PI_Controller_Id ==
  data: e input; V_d_ref output; P input; I_Ts_speed input; reset input; Id0 input; saturation_limit input
function V_d_ref = PI_Controller(e, P, I_Ts_speed, reset, Id0, saturation_limit)
    % PI_Controller: implementa un controllore PI con saturazione e reset.
    % INPUTS:
    % e               -> Errore (input del PI)
    % P               -> Guadagno proporzionale
    % I_Ts_speed      -> Guadagno integrale moltiplicato per Ts (I*Ts_speed)
    % reset           -> Segnale booleano per resettare l'integratore
    % Id0              -> Valore iniziale del riferimento (per l'integratore)
    % saturation_limit -> Limite di saturazione (valore assoluto)
    %
    % OUTPUT:
    % V_d_ref         -> Uscita del controllore PI con saturazione
    
    % Definizione di variabili statiche per la memoria interna del PI
    persistent integrator_state;
    if isempty(integrator_state)
        integrator_state = single(0);  % Inizializza la memoria dell'integratore
    end
    
    % Reset integratore se richiesto
    if reset
        integrator_state = Id0;
    end
    
    % Parte proporzionale
    P_term = P * e;
    
    % Parte integrale (accumulatore)
    integrator_state = integrator_state + I_Ts_speed * e;
    
    % Uscita PI senza saturazione
    V_d_ref_unsat = P_term + integrator_state;
    
    % Saturazione dell'uscita (limite superiore e inferiore)
    V_d_ref = max(min(V_d_ref_unsat, saturation_limit), -saturation_limit);
    
    % Implementazione dell'anti-windup: corregge l'integratore in caso di saturazione
    if V_d_ref ~= V_d_ref_unsat
        integrator_state = integrator_state - I_Ts_speed * e;  % Evita windup
    end
end

== matlab function mcb_pmsm_foc_sensorless_dyno_f28379d/FOC Algorithm Motor 1/Closed Loop/Current_Controllers/PI_Controller_Iq/PI_Controller_Iq ==
  data: e input; V_q_ref output; P input; I_Ts_speed input; reset input; Iq0 input; saturation_limit input
function V_q_ref = PI_Controller(e, P, I_Ts_speed, reset, Iq0, saturation_limit)
    % PI_Controller: implementa un controllore PI con saturazione e reset.
    % INPUTS:
    % e               -> Errore (input del PI)
    % P               -> Guadagno proporzionale
    % I_Ts_speed      -> Guadagno integrale moltiplicato per Ts (I*Ts_speed)
    % reset           -> Segnale booleano per resettare l'integratore
    % Iq0              -> Valore iniziale del riferimento (per l'integratore)
    % saturation_limit -> Limite di saturazione (valore assoluto)
    %
    % OUTPUT:
    % V_q_ref         -> Uscita del controllore PI con saturazione
    
    % Definizione di variabili statiche per la memoria interna del PI
    persistent integrator_state;
    if isempty(integrator_state)
        integrator_state = single(0);  % Inizializza la memoria dell'integratore
    end
    
    % Reset integratore se richiesto
    if reset
        integrator_state = Iq0;
    end
    
    % Parte proporzionale
    P_term = P * e;
    
    % Parte integrale (accumulatore)
    integrator_state = integrator_state + I_Ts_speed * e;
    
    % Uscita PI senza saturazione
    V_q_ref_unsat = P_term + integrator_state;
    
    % Saturazione dell'uscita (limite superiore e inferiore)
    V_q_ref = max(min(V_q_ref_unsat, saturation_limit), -saturation_limit);
    
    % Implementazione dell'anti-windup: corregge l'integratore in caso di saturazione
    if V_q_ref ~= V_q_ref_unsat
        integrator_state = integrator_state - I_Ts_speed * e;  % Evita windup
    end
end

== matlab function mcb_pmsm_foc_sensorless_dyno_f28379d/FOC Algorithm Motor 2/Closed loop/Current_Controllers/PI_Controller_Iq/PI_Controller_Iq ==
  data: e input; V_q_ref output; P input; I_Ts_speed input; reset input; Iq0 input; saturation_limit input
function V_q_ref = PI_Controller(e, P, I_Ts_speed, reset, Iq0, saturation_limit)
    % PI_Controller: implementa un controllore PI con saturazione e reset.
    % INPUTS:
    % e               -> Errore (input del PI)
    % P               -> Guadagno proporzionale
    % I_Ts_speed      -> Guadagno integrale moltiplicato per Ts (I*Ts_speed)
    % reset           -> Segnale booleano per resettare l'integratore
    % Iq0              -> Valore iniziale del riferimento (per l'integratore)
    % saturation_limit -> Limite di saturazione (valore assoluto)
    %
    % OUTPUT:
    % V_q_ref         -> Uscita del controllore PI con saturazione
    
    % Definizione di variabili statiche per la memoria interna del PI
    persistent integrator_state;
    if isempty(integrator_state)
        integrator_state = single(0);  % Inizializza la memoria dell'integratore
    end
    
    % Reset integratore se richiesto
    if reset
        integrator_state = Iq0;
    end
    
    % Parte proporzionale
    P_term = P * e;
    
    % Parte integrale (accumulatore)
    integrator_state = integrator_state + I_Ts_speed * e;
    
    % Uscita PI senza saturazione
    V_q_ref_unsat = P_term + integrator_state;
    
    % Saturazione dell'uscita (limite superiore e inferiore)
    V_q_ref = max(min(V_q_ref_unsat, saturation_limit), -saturation_limit);
    
    % Implementazione dell'anti-windup: corregge l'integratore in caso di saturazione
    if V_q_ref ~= V_q_ref_unsat
        integrator_state = integrator_state - I_Ts_speed * e;  % Evita windup
    end
end

== matlab function mcb_pmsm_foc_sensorless_dyno_f28379d/Speed Control/PI_Controller_Speed/MATLAB Function1 ==
  data: error input; ISE output; Ts input; IAE output; ITAE output
function [ISE,IAE,ITAE] = computeIndices(error, Ts)
    persistent t;
    persistent old_index;

    if isempty(t)
        t=single(0);
    end
    if isempty(old_index)
        old_index.ISE = single(0);
        old_index.IAE = single(0);
        old_index.ITAE = single(0);
    end
    ISE = old_index.ISE + (error^2) * Ts;
    IAE = old_index.IAE + abs(error) * Ts;
    ITAE = old_index.ITAE + t * abs(error) * Ts;
    disp(t)
    if t>=5.999
        assignin('base', 'ISE', ISE);
        assignin('base', 'IAE', IAE);
        assignin('base', 'ITAE', ITAE);
    else
        t=t+Ts;
        old_index.ISE=ISE;
        old_index.IAE=IAE;
        old_index.ITAE=ITAE;
    end
end
